simulink model "PO6x6"  (R2023b)
settings: Solver=VariableStepAuto  StartTime=0.0  StopTime=0.01  RelTol=1e-3
libraries: spsDiodeLib x36, spsPVArrayLib x36, spsSeriesRLCBranchLib x4, spsCurrentMeasurementLib x1, spsMosfetLib x1, slpidlib x1, simulink x1, spsVoltageMeasurementLib x1, sps_lib x1
settings Model: Creator=ASUS  LastModifiedBy=ASUS

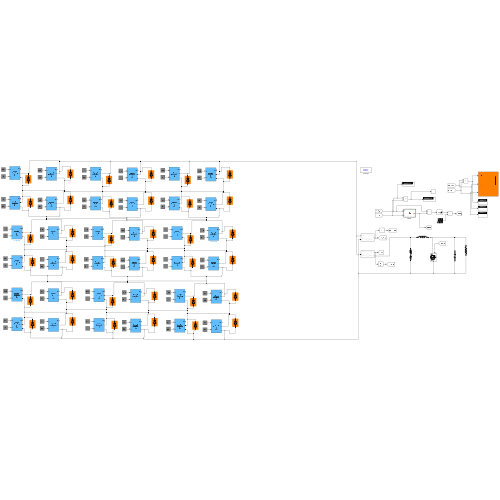
[thumbnail: Simulink's stored preview of the top-level diagram]
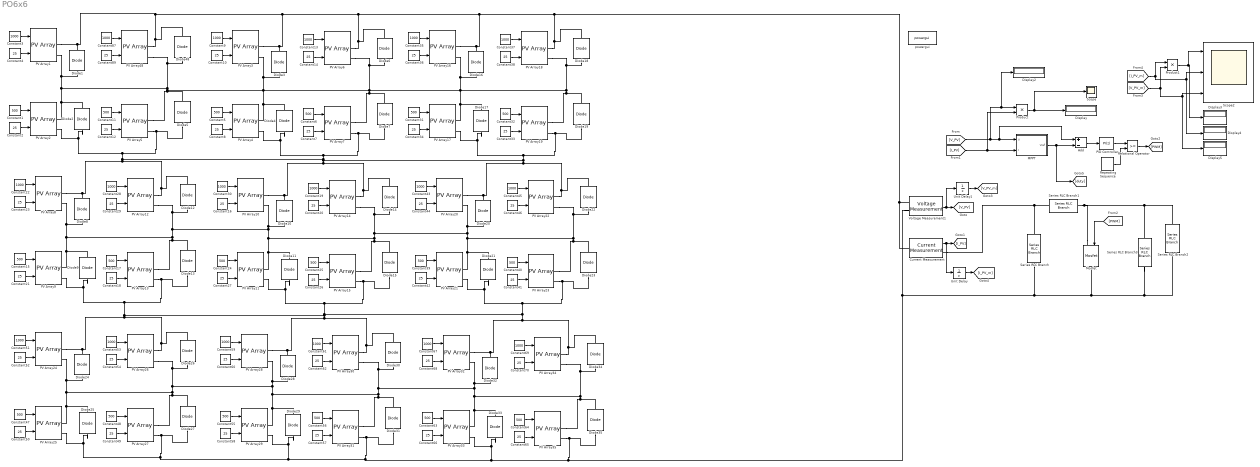
== system PO6x6 ==
  Add : Sum  Inputs=+-
  Constant{1,5..6,11,15,17,24..25,31..32,39..40,47..48,55..56,63..64} (18 alike) : Constant  Value=500
  Constant{2,4,7..8,10,12,14,16,18,20..21,23,26..27,29,33..34,36,38,41..42,44,46,49..50,52,54,57..58,60,62,65..66,68,70,89} (36 alike) : Constant  Value=25
  Constant{3,9,13,19,22,28,30,35,37,43,45,51,53,59,61,67,69,87} (18 alike) : Constant  Value=1000
  Current Measurement : spsCurrentMeasurementLib/Current Measurement  PhasorSimulation=off  OutputType=Complex  PSBequivalent=0
  Diode{1..35,48} (36 alike) : spsDiodeLib/Diode  Ron=0.001  Lon=0  Vf=0.8  IC=0  UseSnubber=0  Rs=inf  Cs=0  Measurements=off
  Display{,2..5} (5 alike) : Display
  MPPT : MATLAB Function  TreatAsAtomicUnit=on
  Mosfet : spsMosfetLib/Mosfet  Ron=0.1  Lon=0  Rd=0.01  Vfd=0  IC=0  Rs=1e5  Cs=inf  Measurements=off
  PID Controller : slpidlib/PID Controller  Controller=PI  Form=Parallel  TimeDomain=Discrete-time  UseExternalTs=off  SampleTime=500e-6  IntegratorMethod=Forward Euler  FilterMethod=Forward Euler  ControllerParametersSource=internal  P=0.7  I=10  UseKiTs=off  D=0  N=100  UseFilter=on  TunerSelectOption=Transfer Function Based (PID Tuner App)  InitialConditionSource=internal  InitialConditionForIntegrator=0.54  InitialConditionForFilter=0  DifferentiatorICPrevScaledInput=0  ExternalReset=none  TrackingMode=off  Kt=1  LimitOutput=on  SatLimitsSource=internal  UpperSaturationLimit=0.95  LowerSaturationLimit=0.1  LinearizeAsGain=on  AntiWindupMode=none  Kb=1  LimitIntegrator=off  UpperIntegratorSaturationLimit=inf  LowerIntegratorSaturationLimit=-inf  POutMin=[]  POutMax=[]  IOutMin=[]  IOutMax=[]  DOutMin=[]  DOutMax=[]  NOutMin=[]  NOutMax=[]  SumOutMin=[]  SumOutMax=[]  SaturationOutMin=[]  SaturationOutMax=[]  PParamMin=[]  PParamMax=[]  IParamMin=[]  IParamMax=[]  DParamMin=[]  DParamMax=[]  NParamMin=[]  NParamMax=[]  KbParamMin=[]  KbParamMax=[]  KtParamMin=[]  KtParamMax=[]  KbOutMin=[]  KbOutMax=[]  KtOutMin=[]  KtOutMax=[]  IntegratorOutMin=[]  IntegratorOutMax=[]  FilterOutMin=[]  FilterOutMax=[]  SumI1OutMin=[]  SumI1OutMax=[]  SumI2OutMin=[]  SumI2OutMax=[]  SumI3OutMin=[]  SumI3OutMax=[]  SumI4OutMin=[]  SumI4OutMax=[]  SumDOutMin=[]  SumDOutMax=[]  DifferentiatorOutMin=[]  DifferentiatorOutMax=[]  FilterDiffOutCoefMin=[]  FilterDiffOutCoefMax=[]  ReciprocalOutMin=[]  ReciprocalOutMax=[]  SumDenOutMin=[]  SumDenOutMax=[]  SumNumOutMin=[]  SumNumOutMax=[]  DivideOutMin=[]  DivideOutMax=[]  UdiffTsProdOutMin=[]  UdiffTsProdOutMax=[]  NTsProdOutMin=[]  NTsProdOutMax=[]  UintegralTsProdOutMin=[]  UintegralTsProdOutMax=[]  UngainTsProdOutMin=[]  UngainTsProdOutMax=[]  ClampingZeroOutDataTypeStr=Inherit: Inherit via back propagation  ClampingZeroOutMin=[]  ClampingZeroOutMax=[]  FilterDenConstantOutDataTypeStr=Inherit: Inherit via back propagation  FilterDenConstantOutMin=[]  FilterDenConstantOutMax=[]  PCopyOutDataTypeStr=Inherit: Inherit via back propagation  PCopyOutMin=[]  PCopyOutMax=[]  NCopyOutDataTypeStr=Inherit: Inherit via back propagation  NCopyOutMin=[]  NCopyOutMax=[]  IntegratorContinuousStateAttributes=''  IntegratorStateMustResolveToSignalObject=off  IntegratorRTWStateStorageClass=Auto  FilterContinuousStateAttributes=''  FilterStateMustResolveToSignalObject=off  FilterRTWStateStorageClass=Auto  ParallelPVariant=InternalParameters  IdealPVariant=Disabled  IVariant=InternalParameters  DVariant=Disabled  IntegratorVariant=Discrete  SatVariant=Enabled  AWVariant=Passthrough  PCopyVariant=Disabled  TRVariant=Disabled  FdbkBlocksVariant=Forward  IdealPFdbkVariant=Disabled  SatFdbkVariant=Disabled  DerivativeFilterVariant=Disabled  NVariant=Disabled  NCopyVariant=Disabled_SignalSpec  FilterICVariant=Disabled  IntegratorICVariant=InternalICs  ExternalResetVariant=Disabled  TRSumVariant=Passthrough  SumFdbkVariant=Disabled  SumVariant=Sum_PI  TsampFilterVariant=InternalTs  TsampNgainVariant=Passthrough  TsampIntegralVariant=Disabled_SignalSpec  ExternalSaturationOutDataTypeStr=Inherit: Same as second input
  PV Array{1..35,48} (36 alike) : spsPVArrayLib/PV Array  Npar=1  Nser=1  PlotType=one module @ 25 deg.C & specified irradiances  S_vec="[ 1000  500  100 ]"  Temp_C_vec="[ 45 25  ]"  ModuleName=BIPV BIPV054-S86  PlotWhenSelected=off  Pm=53.976  Ncell=14  Voc=8.87  Isc=8.22  Vm=6.92  Im=7.8  beta_Voc_pc=-0.36  alpha_Isc_pc=0.06  beta_Voc=-0.031932  alpha_Isc=0.004932  IL=8.263  I0=2.8018e-10  nI=1.0231  Rsh=333.8433  Rs=0.11548  RobustModel=off  RobustCellTemperature=313.3991  BAL=off  Tc=1e-6  Tfilter=5e-5
  Product : Product
  Product1 : Product
  Relational Operator : RelationalOperator  OutDataTypeStr=boolean  RndMeth=Simplest  InputSameDT=off
  Repeating Sequence : simulink/Sources/Repeating Sequence  rep_seq_t=[0 0.0002]  rep_seq_y=[0 1]
  Scope : Scope
  Scope2 : Scope  NumInputPorts=3
  Series RLC Branch : spsSeriesRLCBranchLib/Series RLC Branch  LConnTagsString=__new0  RConnTagsString=__new0  BranchType=RC  Resistance=0.0001  Inductance=1e-3  SetiL0=off  InitialCurrent=0  Capacitance=968e-6  Setx0=off  InitialVoltage=0  Measurements=None
  Series RLC Branch1 : spsSeriesRLCBranchLib/Series RLC Branch  LConnTagsString=__new0  RConnTagsString=__new0  BranchType=L  Resistance=0.0001  Inductance=1.6e-3  SetiL0=off  InitialCurrent=0  Capacitance=968e-6  Setx0=off  InitialVoltage=0  Measurements=None
  Series RLC Branch2 : spsSeriesRLCBranchLib/Series RLC Branch  LConnTagsString=__new0  RConnTagsString=__new0  BranchType=R  Resistance=4  Inductance=1e-3  SetiL0=off  InitialCurrent=0  Capacitance=968e-6  Setx0=off  InitialVoltage=0  Measurements=None
  Series RLC Branch3 : spsSeriesRLCBranchLib/Series RLC Branch  LConnTagsString=__new0  RConnTagsString=__new0  BranchType=C  Resistance=0.0001  Inductance=1e-3  SetiL0=off  InitialCurrent=0  Capacitance=3300e-6  Setx0=off  InitialVoltage=0  Measurements=None
  Unit Delay : UnitDelay  SampleTime=-1  HasFrameUpgradeWarning=on
  Unit Delay1 : UnitDelay  SampleTime=-1  HasFrameUpgradeWarning=on
  Voltage Measurement1 : spsVoltageMeasurementLib/Voltage Measurement  PhasorSimulation=off  OutputType=Complex  PSBequivalent=0
  powergui : sps_lib/powergui  Priority=1  SimulationMode=Discrete  SampleTime=5e-6  frequency=60  Iterations=50  frequencyindice=0  Pbase=100e6  ErrMax=1e-4  UnitsV=kV  UnitsW=MW  buscounter=0  FunctionMessages=off  echomessages=off  EnableUseOfTLC=off  CurrentSourceSwitches=off  DisableSnubberDevices=off  DisableRonSwitches=off  DisableVfSwitches=off  DisplayEquations=off  AutomaticDiscreteSolvers=off  SolverType=Tustin/Backward Euler (TBE)  Interpol=off  ExternalGateDelay=off  methode=off  Ts=100  x0status=blocks  SPID=on  SwTol=0  HookPort=off  NonlinearTolerance=1e-4  nMaxIteration=100  ContinueOnMaxIteration=off  RestoreLinks=warning  ResistiveCurrentMeasurement=off  Frange=[0:2:500]  Ylog=off  Xlog=on  ShowGrid=off  save=off  variable=ZData  structure=0  ZoomFFT=off  StartTime=0.0  cycles=1  DisplayStyle=1  fundamental=60  FreqAxis=off  MaxFrequency=1000  frequencyindicesteady=1  RmsSteady=1  display=off
  wires:
  Product/1 -> Scope/1, Display/1
  [PWM] -> Mosfet/1
  Repeating Sequence/1 -> Relational Operator/2
  MPPT/1(Vref) -> [duty], Add/2
  [V_PV] -> Display2/1, Product/1, Add/1, MPPT/1(V)
  Add/1 -> PID Controller/1
  Relational Operator/1 -> [PWM]
  Current Measurement/1 -> Unit Delay/1, [I_PV]
  PID Controller/1 -> Relational Operator/1
  [I_PV] -> MPPT/2(I), Product/2
  Constant89/1 -> PV Array48/2
  Constant87/1 -> PV Array48/1
  Constant12/1 -> PV Array5/2
  Constant11/1 -> PV Array5/1
  Constant3/1 -> PV Array1/1
  Constant4/1 -> PV Array1/2
  Constant1/1 -> PV Array2/1
  Constant2/1 -> PV Array2/2
  Voltage Measurement1/1 -> Unit Delay1/1, [V_PV]
  Unit Delay1/1 -> [V_PV_m]
  Unit Delay/1 -> [I_PV_m]
  [I_PV_m] -> Product1/1, Display4/1, Scope2/2
  [V_PV_m] -> Product1/2, Display5/1, Scope2/3
  Product1/1 -> Scope2/1, Display3/1
  Constant8/1 -> PV Array4/2
  Constant13/1 -> PV Array6/1
  Constant6/1 -> PV Array7/1
  Constant7/1 -> PV Array7/2
  Constant5/1 -> PV Array4/1
  Constant10/1 -> PV Array3/2
  Constant14/1 -> PV Array6/2
  Constant9/1 -> PV Array3/1
  Constant26/1 -> PV Array15/2
  Constant19/1 -> PV Array14/1
  Constant20/1 -> PV Array14/2
  Constant16/1 -> PV Array10/2
  Constant24/1 -> PV Array11/1
  Constant30/1 -> PV Array10/1
  Constant25/1 -> PV Array15/1
  Constant21/1 -> PV Array9/2
  Constant28/1 -> PV Array12/1
  Constant17/1 -> PV Array13/1
  Constant18/1 -> PV Array13/2
  Constant27/1 -> PV Array11/2
  Constant15/1 -> PV Array9/1
  Constant23/1 -> PV Array8/2
  Constant29/1 -> PV Array12/2
  Constant22/1 -> PV Array8/1
  Constant34/1 -> PV Array17/2
  Constant37/1 -> PV Array18/1
  Constant32/1 -> PV Array19/1
  Constant33/1 -> PV Array19/2
  Constant31/1 -> PV Array17/1
  Constant36/1 -> PV Array16/2
  Constant38/1 -> PV Array18/2
  Constant35/1 -> PV Array16/1
  Constant42/1 -> PV Array21/2
  Constant45/1 -> PV Array22/1
  Constant40/1 -> PV Array23/1
  Constant41/1 -> PV Array23/2
  Constant39/1 -> PV Array21/1
  Constant44/1 -> PV Array20/2
  Constant46/1 -> PV Array22/2
  Constant43/1 -> PV Array20/1
  Constant50/1 -> PV Array25/2
  Constant53/1 -> PV Array26/1
  Constant48/1 -> PV Array27/1
  Constant49/1 -> PV Array27/2
  Constant47/1 -> PV Array25/1
  Constant52/1 -> PV Array24/2
  Constant54/1 -> PV Array26/2
  Constant51/1 -> PV Array24/1
  Constant58/1 -> PV Array29/2
  Constant61/1 -> PV Array30/1
  Constant56/1 -> PV Array31/1
  Constant57/1 -> PV Array31/2
  Constant55/1 -> PV Array29/1
  Constant60/1 -> PV Array28/2
  Constant62/1 -> PV Array30/2
  Constant59/1 -> PV Array28/1
  Constant66/1 -> PV Array33/2
  Constant69/1 -> PV Array34/1
  Constant64/1 -> PV Array35/1
  Constant65/1 -> PV Array35/2
  Constant63/1 -> PV Array33/1
  Constant68/1 -> PV Array32/2
  Constant70/1 -> PV Array34/2
  Constant67/1 -> PV Array32/1
  connections:
  PV Array27/RConn2 -- Diode25/LConn1 -- PV Array25/RConn2 -- Voltage Measurement1/LConn2 -- Series RLC Branch/RConn1 -- Mosfet/RConn1 -- Series RLC Branch2/RConn1 -- Series RLC Branch3/RConn1 -- Diode35/LConn1 -- PV Array35/RConn2 -- Diode33/LConn1 -- PV Array33/RConn2 -- Diode31/LConn1 -- PV Array31/RConn2 -- Diode29/LConn1 -- PV Array29/RConn2 -- Diode27/LConn1
  Series RLC Branch/LConn1 -- Current Measurement/RConn1 -- Series RLC Branch1/RConn1
  Mosfet/LConn1 -- Series RLC Branch2/LConn1 -- Series RLC Branch3/LConn1 -- Series RLC Branch1/LConn1
  Diode1/RConn1 -- PV Array6/RConn1 -- Diode6/RConn1 -- Current Measurement/LConn1 -- Voltage Measurement1/LConn1 -- PV Array18/RConn1 -- Diode18/RConn1 -- Diode16/RConn1 -- PV Array16/RConn1 -- Diode3/RConn1 -- PV Array3/RConn1 -- PV Array48/RConn1 -- Diode48/RConn1 -- PV Array1/RConn1
  PV Array1/RConn2 -- PV Array16/RConn2 -- Diode16/LConn1 -- Diode17/RConn1 -- PV Array17/RConn1 -- PV Array19/RConn1 -- Diode19/RConn1 -- PV Array18/RConn2 -- Diode18/LConn1 -- PV Array7/RConn1 -- Diode7/RConn1 -- PV Array6/RConn2 -- Diode6/LConn1 -- PV Array3/RConn2 -- Diode3/LConn1 -- Diode4/RConn1 -- PV Array4/RConn1 -- PV Array5/RConn1 -- Diode5/RConn1 -- PV Array48/RConn2 -- Diode48/LConn1 -- Diode2/RConn1 -- PV Array2/RConn1 -- Diode1/LConn1
  Diode2/LConn1 -- PV Array2/RConn2 -- PV Array12/RConn1 -- Diode12/RConn1 -- Diode8/RConn1 -- PV Array8/RConn1 -- PV Array22/RConn1 -- Diode22/RConn1 -- Diode20/RConn1 -- PV Array20/RConn1 -- Diode19/LConn1 -- PV Array19/RConn2 -- Diode17/LConn1 -- PV Array17/RConn2 -- PV Array14/RConn1 -- Diode14/RConn1 -- Diode10/RConn1 -- PV Array10/RConn1 -- Diode7/LConn1 -- PV Array7/RConn2 -- Diode4/LConn1 -- PV Array4/RConn2 -- Diode5/LConn1 -- PV Array5/RConn2
  Diode12/LConn1 -- PV Array14/RConn2 -- Diode14/LConn1 -- PV Array20/RConn2 -- Diode20/LConn1 -- Diode21/RConn1 -- PV Array21/RConn1 -- PV Array23/RConn1 -- Diode23/RConn1 -- PV Array22/RConn2 -- Diode22/LConn1 -- PV Array15/RConn1 -- Diode15/RConn1 -- Diode11/RConn1 -- PV Array11/RConn1 -- PV Array10/RConn2 -- Diode10/LConn1 -- PV Array8/RConn2 -- Diode8/LConn1 -- Diode9/RConn1 -- PV Array9/RConn1 -- PV Array13/RConn1 -- Diode13/RConn1 -- PV Array12/RConn2
  PV Array13/RConn2 -- Diode15/LConn1 -- PV Array15/RConn2 -- Diode11/LConn1 -- PV Array11/RConn2 -- PV Array34/RConn1 -- Diode34/RConn1 -- Diode32/RConn1 -- PV Array32/RConn1 -- Diode23/LConn1 -- PV Array23/RConn2 -- Diode21/LConn1 -- PV Array21/RConn2 -- PV Array30/RConn1 -- Diode30/RConn1 -- Diode28/RConn1 -- PV Array28/RConn1 -- PV Array26/RConn1 -- Diode26/RConn1 -- Diode24/RConn1 -- PV Array24/RConn1 -- Diode9/LConn1 -- PV Array9/RConn2 -- Diode13/LConn1
  Diode26/LConn1 -- Diode29/RConn1 -- PV Array29/RConn1 -- PV Array30/RConn2 -- Diode30/LConn1 -- Diode33/RConn1 -- PV Array33/RConn1 -- PV Array35/RConn1 -- Diode35/RConn1 -- PV Array34/RConn2 -- Diode34/LConn1 -- PV Array32/RConn2 -- Diode32/LConn1 -- PV Array31/RConn1 -- Diode31/RConn1 -- PV Array28/RConn2 -- Diode28/LConn1 -- PV Array24/RConn2 -- Diode24/LConn1 -- Diode25/RConn1 -- PV Array25/RConn1 -- PV Array27/RConn1 -- Diode27/RConn1 -- PV Array26/RConn2

== matlab function PO6x6/MPPT ==
  data: V input; Vref output; I input
function Vref = MPPT(V,I)

Vrefmax = 450;
Vrefmin = 0;
Vrefinit = 400;
deltaVref =1;
persistent Volt Polt Vreffolt;

dataType = 'double';

if isempty (Volt)
    Volt = 0;
    Polt = 0;
    Vreffolt = Vrefinit;
end

P=V*I;
dV = V-Volt;
dP = P-Polt;

if dP ~= 0
    if dP < 0
        if dV < 0
            Vref = Vreffolt + deltaVref;
        else
            Vref = Vreffolt - deltaVref;
        end
    else
        if dV < 0
            Vref = Vreffolt - deltaVref;
        else
            Vref = Vreffolt + deltaVref;
        end
    end
else
    Vref = Vreffolt;
end

if Vref >= Vrefmax || Vref <= Vrefmin
    Vref = Vreffolt;
end

Vreffolt = Vref;
Volt = V;
Pout = P;
